simulink model "PROYECTO_FINAL_TEORICO"  (R2019a)
settings: Solver=VariableStepAuto  StartTime=0.0  StopTime=50  RelTol=1e-3
values from neighbouring files (symbols this model uses):
  P0 = B(1)    [controlalgebraicoposorden4.m]
  P1 = B(3)    [controlalgebraicoposorden4.m]
  P2 = B(5)    [controlalgebraicoposorden4.m]
  P3 = B(7)    [controlalgebraicoposorden4.m]
  Q0 = B(2)    [controlalgebraicoposorden4.m]
  Q1 = B(4)    [controlalgebraicoposorden4.m]
  Q2 = B(6)    [controlalgebraicoposorden4.m]
  Q3 = B(8)    [controlalgebraicoposorden4.m]
undefined symbols (not defined in the file or in its folder): DiscIntNeverNeededParam
libraries: simulink x6
settings Model: Creator=STEVEN  LastModifiedBy=isabella_mar.lopez

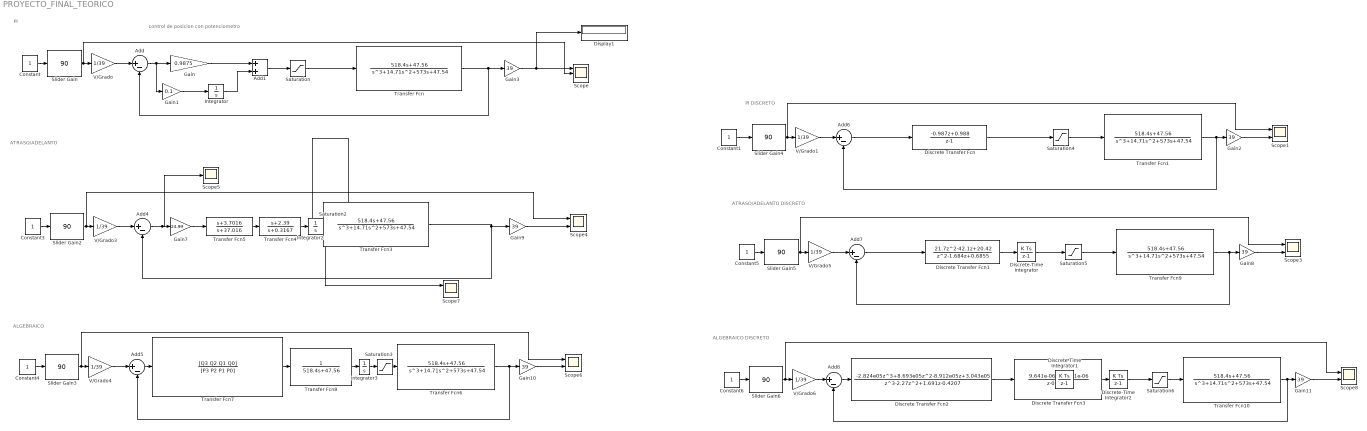
== system PROYECTO_FINAL_TEORICO ==
  note: ALGEBRAICO DISCRETO
  note: ATRASO/ADELANTO DISCRETO
  note: PI DISCRETO
  note: ALGEBRAICO
  note: ATRASO/ADELANTO
  note: PI
  note: control de posicion con potenciometro
  Add{,4..8} (6 alike) : Sum  Inputs=|+-
  Add1 : Sum
  Constant{,1,3..6} (6 alike) : Constant
  Discrete Transfer Fcn : DiscreteTransferFcn  Numerator=[-0.987 0.988]  Denominator=[1 -1]  SampleTime=0.01
  Discrete Transfer Fcn1 : DiscreteTransferFcn  Numerator=[21.7 -42.1 20.42]  Denominator=[1 -1.684 0.6855]  SampleTime=0.01
  Discrete Transfer Fcn2 : DiscreteTransferFcn  Numerator="[-2.824e05  8.693e05 -8.912e05 3.043e05]"  Denominator=[1 -2.27 1.691 -0.4207]  SampleTime=0.01
  Discrete Transfer Fcn3 : DiscreteTransferFcn  Numerator=[9.641e-06 9.641e-06]  Denominator=[1 -0.9991]  SampleTime=0.01
  Discrete-Time Integrator : DiscreteIntegrator  SampleTime=0.01  ICPrevOutput=DiscIntNeverNeededParam  ICPrevScaledInput=DiscIntNeverNeededParam
  Discrete-Time Integrator1 : DiscreteIntegrator  SampleTime=-1  ICPrevOutput=DiscIntNeverNeededParam  ICPrevScaledInput=DiscIntNeverNeededParam
  Discrete-Time Integrator2 : DiscreteIntegrator  SampleTime=0.01  ICPrevOutput=DiscIntNeverNeededParam  ICPrevScaledInput=DiscIntNeverNeededParam
  Display1 : Display
  Gain : Gain  Gain=0.9875
  Gain1 : Gain  Gain=0.1
  Gain{2..3,8..11} (6 alike) : Gain  Gain=39
  Gain7 : Gain  Gain=24.99
  Integrator : Integrator
  Integrator2 : Integrator
  Integrator3 : Integrator
  Saturation : Saturate  UpperLimit=10  LowerLimit=-10
  Saturation2 : Saturate  UpperLimit=10  LowerLimit=-10
  Saturation3 : Saturate  UpperLimit=5  LowerLimit=-5
  Saturation4 : Saturate  UpperLimit=5  LowerLimit=-5
  Saturation5 : Saturate  UpperLimit=5  LowerLimit=-5
  Saturation6 : Saturate  UpperLimit=10  LowerLimit=-10
  Scope : Scope  NumInputPorts=3
  Scope{1,3..4,6..8} (6 alike) : Scope  NumInputPorts=2
  Scope5 : Scope
  Slider Gain{,2..6} (6 alike) : simulink/Math Operations/Slider Gain  gain=90  low=-180  high=180
  Transfer Fcn{,1,3,6,9..10} (6 alike) : TransferFcn  Numerator=[518.4 47.56]  Denominator=[1 14.71 573 47.54]
  Transfer Fcn4 : TransferFcn  Numerator=[1 2.39]  Denominator=[1 0.3167]
  Transfer Fcn5 : TransferFcn  Numerator=[1 3.7016]  Denominator=[1 37.016]
  Transfer Fcn7 : TransferFcn  Numerator=[Q3 Q2 Q1 Q0]  Denominator=[P3 P2 P1 P0]
  Transfer Fcn8 : TransferFcn  Numerator=1  Denominator=[518.4 47.56]
  V/Grado{,1,3..6} (6 alike) : Gain  Gain=1/39
  wires:
  Add1/1 -> Saturation/1
  Transfer Fcn/1 -> Gain3/1, Add/2
  V/Grado/1 -> Add/1
  Slider Gain/1 -> Scope/2, V/Grado/1
  Integrator/1 -> Add1/2
  Gain1/1 -> Integrator/1
  Add/1 -> Gain1/1, Gain/1
  Saturation/1 -> Transfer Fcn/1
  Constant/1 -> Slider Gain/1
  Gain/1 -> Add1/1
  Gain3/1 -> Display1/1, Scope/1
  Slider Gain2/1 -> Scope4/1, V/Grado3/1
  Gain9/1 -> Scope4/2
  Transfer Fcn4/1 -> Integrator2/1
  V/Grado3/1 -> Add4/1
  Transfer Fcn3/1 -> Add4/2, Gain9/1
  Constant3/1 -> Slider Gain2/1
  Saturation2/1 -> Transfer Fcn3/1
  Transfer Fcn5/1 -> Transfer Fcn4/1
  Add4/1 -> Scope5/1, Gain7/1
  Gain7/1 -> Transfer Fcn5/1
  Integrator2/1 -> Scope7/1, Saturation2/1
  Constant4/1 -> Slider Gain3/1
  V/Grado4/1 -> Add5/1
  Slider Gain3/1 -> Scope6/1, V/Grado4/1
  Transfer Fcn6/1 -> Add5/2, Gain10/1
  Add5/1 -> Transfer Fcn7/1
  Gain10/1 -> Scope6/2
  Transfer Fcn7/1 -> Transfer Fcn8/1
  Saturation3/1 -> Transfer Fcn6/1
  Saturation4/1 -> Transfer Fcn1/1
  Add6/1 -> Discrete Transfer Fcn/1
  Gain2/1 -> Scope1/2
  V/Grado1/1 -> Add6/1
  Constant1/1 -> Slider Gain4/1
  Discrete Transfer Fcn/1 -> Saturation4/1
  Slider Gain4/1 -> Scope1/1, V/Grado1/1
  Transfer Fcn1/1 -> Add6/2, Gain2/1
  V/Grado5/1 -> Add7/1
  Transfer Fcn9/1 -> Add7/2, Gain8/1
  Discrete Transfer Fcn1/1 -> Discrete-Time Integrator/1
  Slider Gain5/1 -> Scope3/1, V/Grado5/1
  Constant5/1 -> Slider Gain5/1
  Gain8/1 -> Scope3/2
  Add7/1 -> Discrete Transfer Fcn1/1
  Saturation5/1 -> Transfer Fcn9/1
  V/Grado6/1 -> Add8/1
  Transfer Fcn10/1 -> Add8/2, Gain11/1
  Slider Gain6/1 -> Scope8/1, V/Grado6/1
  Constant6/1 -> Slider Gain6/1
  Gain11/1 -> Scope8/2
  Saturation6/1 -> Transfer Fcn10/1
  Discrete-Time Integrator/1 -> Saturation5/1
  Add8/1 -> Discrete Transfer Fcn2/1
  Discrete Transfer Fcn2/1 -> Discrete Transfer Fcn3/1
  Discrete Transfer Fcn3/1 -> Discrete-Time Integrator2/1
  Discrete-Time Integrator2/1 -> Saturation6/1
  Transfer Fcn8/1 -> Integrator3/1
  Integrator3/1 -> Saturation3/1
